simulink model "DISCON_NREL5MW"  (R2016b)
settings: Solver=FixedStepDiscrete  StartTime=0.0  StopTime=inf  FixedStep=Control.DT  RelTol=1e-3
values from neighbouring files (symbols this model uses):
  CertificationSettings =     [Parameters.mat]
  Control =     [Parameters.mat]
  Drivetrain =     [Parameters.mat]
  P_InitAngle = 0.106    [Parameters.mat]
  T_GenSpeedInit = 1104.83    [Parameters.mat]
undefined symbols (not defined in the file or in its folder): DiscIntNeverNeededParam, dLP
settings Model: Creator=evansolingen  LastModifiedBy=sebastiaanmuld
settings DataIOCC: LimitDataPoints=on  SaveFormat=Array  SignalLoggingSaveFormat=ModelDataLogs  SaveOutput=off  SignalLogging=off  SaveTime=off
settings OptimizationCC: ExpressionDepthLimit=2147483647  LifeSpan=inf
settings DebuggingCC: UnderspecifiedInitializationDetection=Classic  MergeDetectMultiDrivingBlocksExec=none  SolverPrmCheckMsg=warning  MultiTaskDSMMsg=warning  MultiTaskCondExecSysMsg=none  FcnCallInpInsideContextMsg=warning  AllowSymbolicDim=off  StateNameClashWarn=warning  SFUnexpectedBacktrackingDiag=warning  SFNoUnconditionalDefaultTransitionDiag=warning  SFExecutionAtInitializationDiag=none
settings HardwareCC: ProdBitPerPointer=32  ProdBitPerSizeT=32  ProdBitPerPtrDiffT=32  ProdLargestAtomicFloat=None  ProdIntDivRoundTo=Undefined  ProdEndianess=Unspecified  ProdWordSize=32  ProdHWDeviceType=32-bit Generic
settings ModelReferenceCC: UpdateModelReferenceTargets=Force  PropagateSignalLabelsOutOfModel=off
settings SFSimCC: SimParseCustomCode=off  SimBuildMode=sf_make_clean
settings RTWCC: SystemTargetFile=discon.tlc  TemplateMakefile=discon_vc.tmf  Description=DISCON DLL Target (for use with GH BLADED)
settings GRTTargetCC: TargetLangStandard=C89/C90 (ANSI)  GeneratePreprocessorConditionals=Disable all  CombineOutputUpdateFcns=off  GRTInterface=on  UseToolchainInfoCompliant=off  ExtModeMexFile=noextcomm
settings ConfigComp: CovMetricSettings=dw  CovHtmlReporting=on  CovSaveCumulativeToWorkspaceVar=on  CovSaveSingleToWorkspaceVar=on  CovExternalEMLEnable=off

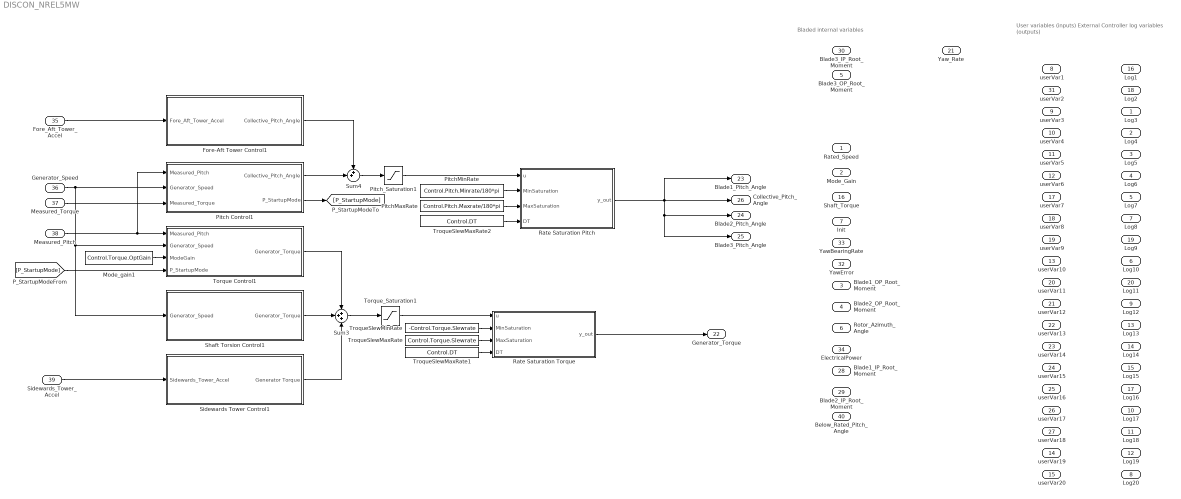
== system DISCON_NREL5MW ==
  note: Bladed internal variables
  note: User variables (inputs)
      | External Controller log variables (outputs)
  Rated_Speed : Inport  PortDimensions=1
  Mode_Gain : Inport  Port=2  PortDimensions=1
  Blade1_OP_Root_Moment : Inport  Port=3  PortDimensions=1
  Blade2_OP_Root_Moment : Inport  Port=4  PortDimensions=1
  Blade3_OP_Root_Moment : Inport  Port=5  PortDimensions=1
  Rotor_Azimuth_Angle : Inport  Port=6  PortDimensions=1
  Init : Inport  Port=7  PortDimensions=1
  userVar1 : Inport  Port=8  PortDimensions=1
  userVar3 : Inport  Port=9  PortDimensions=1
  userVar4 : Inport  Port=10  PortDimensions=1
  userVar5 : Inport  Port=11  PortDimensions=1
  userVar6 : Inport  Port=12  PortDimensions=1
  userVar10 : Inport  Port=13  PortDimensions=1
  userVar19 : Inport  Port=14  PortDimensions=1
  userVar20 : Inport  Port=15  PortDimensions=1
  Shaft_Torque : Inport  Port=16  PortDimensions=1
  userVar7 : Inport  Port=17  PortDimensions=1
  userVar8 : Inport  Port=18  PortDimensions=1
  userVar9 : Inport  Port=19  PortDimensions=1
  userVar11 : Inport  Port=20  PortDimensions=1
  userVar12 : Inport  Port=21  PortDimensions=1
  userVar13 : Inport  Port=22  PortDimensions=1
  userVar14 : Inport  Port=23  PortDimensions=1
  userVar15 : Inport  Port=24  PortDimensions=1
  userVar16 : Inport  Port=25  PortDimensions=1
  userVar17 : Inport  Port=26  PortDimensions=1
  userVar18 : Inport  Port=27  PortDimensions=1
  Blade1_IP_Root_Moment : Inport  Port=28  PortDimensions=1
  Blade2_IP_Root_Moment : Inport  Port=29  PortDimensions=1
  Blade3_IP_Root_Moment : Inport  Port=30  PortDimensions=1
  userVar2 : Inport  Port=31  PortDimensions=1
  YawError : Inport  Port=32  PortDimensions=1
  YawBearingRate : Inport  Port=33  PortDimensions=1
  ElectricalPower : Inport  Port=34  PortDimensions=1
  Fore_Aft_Tower_Accel : Inport  Port=35  PortDimensions=1
  Generator_Speed : Inport  Port=36  PortDimensions=1
  Measured_Torque : Inport  Port=37  PortDimensions=1
  Measured_Pitch : Inport  Port=38  PortDimensions=1
  Sidewards_Tower_Accel : Inport  Port=39  PortDimensions=1
  Below_Rated_Pitch_Angle : Inport  Port=40  PortDimensions=1
  Fore-Aft Tower Control1 : Subsystem
  Mode_gain1 : Constant  Value=Control.Torque.OptGain
  Pitch Control1 : Subsystem
  PitchMaxRate : Constant  Value=Control.Pitch.Maxrate/180*pi
  PitchMinRate : Constant  Value=Control.Pitch.Minrate/180*pi
  Pitch_Saturation1 : Saturate  UpperLimit=Control.Pitch.Max*pi/180  LowerLimit=Control.Pitch.Min*pi/180
  Rate Saturation Pitch : MATLAB Function  TreatAsAtomicUnit=on
  Rate Saturation Torque : MATLAB Function  TreatAsAtomicUnit=on
  Shaft Torsion Control1 : Subsystem
  Sidewards Tower Control1 : Subsystem
  Sum3 : Sum  Inputs=+++
  Sum4 : Sum  Inputs=++|
  Torque Control1 : Subsystem
  Torque_Saturation1 : Saturate  UpperLimit=Control.Torque.Limit  LowerLimit=Control.Torque.Min
  TroqueSlewMaxRate : Constant  Value=Control.Torque.Slewrate
  TroqueSlewMaxRate1 : Constant  Value=Control.DT
  TroqueSlewMaxRate2 : Constant  Value=Control.DT
  TroqueSlewMinRate : Constant  Value=-Control.Torque.Slewrate
  Log3 : Outport  PortDimensions=1
  Log4 : Outport  Port=2  PortDimensions=1
  Log5 : Outport  Port=3  PortDimensions=1
  Log6 : Outport  Port=4  PortDimensions=1
  Log7 : Outport  Port=5  PortDimensions=1
  Log10 : Outport  Port=6  PortDimensions=1
  Log8 : Outport  Port=7  PortDimensions=1
  Log20 : Outport  Port=8  PortDimensions=1
  Log12 : Outport  Port=9  PortDimensions=1
  Log17 : Outport  Port=10  PortDimensions=1
  Log18 : Outport  Port=11  PortDimensions=1
  Log19 : Outport  Port=12  PortDimensions=1
  Log13 : Outport  Port=13  PortDimensions=1
  Log14 : Outport  Port=14  PortDimensions=1
  Log15 : Outport  Port=15  PortDimensions=1
  Log1 : Outport  Port=16  PortDimensions=1
  Log16 : Outport  Port=17  PortDimensions=1
  Log2 : Outport  Port=18  PortDimensions=1
  Log9 : Outport  Port=19  PortDimensions=1
  Log11 : Outport  Port=20  PortDimensions=1
  Yaw_Rate : Outport  Port=21  PortDimensions=1
  Generator_Torque : Outport  Port=22  PortDimensions=1
  Blade1_Pitch_Angle : Outport  Port=23  PortDimensions=1
  Blade2_Pitch_Angle : Outport  Port=24  PortDimensions=1
  Blade3_Pitch_Angle : Outport  Port=25  PortDimensions=1
  Collective_Pitch_Angle : Outport  Port=26  PortDimensions=1
  wires:
  Sidewards_Tower_Accel/1 -> Sidewards Tower Control1/1(Sidewards_Tower_Accel)
  Fore_Aft_Tower_Accel/1 -> Fore-Aft Tower Control1/1(Fore_Aft_Tower_Accel)
  Fore-Aft Tower Control1/1(Collective_Pitch_Angle) -> Sum4/1
  Torque Control1/1(Generator_Torque) -> Sum3/1
  Sidewards Tower Control1/1(Generator Torque) -> Sum3/3
  Measured_Pitch/1 -> Pitch Control1/1(Measured_Pitch), Torque Control1/1(Measured_Pitch)
  Measured_Torque/1 -> Pitch Control1/3(Measured_Torque)
  Shaft Torsion Control1/1(Generator_Torque) -> Sum3/2
  Mode_gain1/1 -> Torque Control1/3(ModeGain)
  Sum3/1 -> Torque_Saturation1/1
  Sum4/1 -> Pitch_Saturation1/1
  Rate Saturation Pitch/1(y_out) -> Blade1_Pitch_Angle/1, Collective_Pitch_Angle/1, Blade3_Pitch_Angle/1, Blade2_Pitch_Angle/1
  PitchMinRate/1 -> Rate Saturation Pitch/2(MinSaturation)
  PitchMaxRate/1 -> Rate Saturation Pitch/3(MaxSaturation)
  Pitch_Saturation1/1 -> Rate Saturation Pitch/1(u)
  Torque_Saturation1/1 -> Rate Saturation Torque/1(u)
  TroqueSlewMinRate/1 -> Rate Saturation Torque/2(MinSaturation)
  TroqueSlewMaxRate/1 -> Rate Saturation Torque/3(MaxSaturation)
  Generator_Speed/1 -> Pitch Control1/2(Generator_Speed), Torque Control1/2(Generator_Speed), Shaft Torsion Control1/1(Generator_Speed)
  [P_StartupMode] -> Torque Control1/4(P_StartupMode)
  Pitch Control1/2(P_StartupMode) -> [P_StartupMode]
  Pitch Control1/1(Collective_Pitch_Angle) -> Sum4/2
  Rate Saturation Torque/1(y_out) -> Generator_Torque/1
  TroqueSlewMaxRate1/1 -> Rate Saturation Torque/4(DT)
  TroqueSlewMaxRate2/1 -> Rate Saturation Pitch/4(DT)

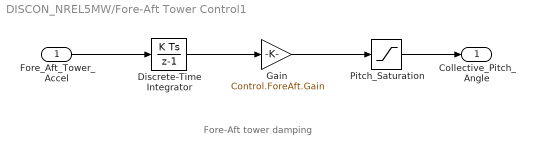
== system DISCON_NREL5MW/Fore-Aft Tower Control1 ==
  note: Fore-Aft tower damping
  Fore_Aft_Tower_Accel : Inport
  Discrete-Time Integrator : DiscreteIntegrator  SampleTime=-1  ICPrevOutput=DiscIntNeverNeededParam  ICPrevScaledInput=DiscIntNeverNeededParam
  Gain : Gain  Gain=Control.ForeAft.Gain
  Pitch_Saturation : Saturate  UpperLimit=Control.ForeAft.MaxPitchAmplitude*pi/180  LowerLimit=-Control.ForeAft.MaxPitchAmplitude*pi/180
  Collective_Pitch_Angle : Outport
  wires:
  Fore_Aft_Tower_Accel/1 -> Discrete-Time Integrator/1
  Pitch_Saturation/1 -> Collective_Pitch_Angle/1
  Discrete-Time Integrator/1 -> Gain/1
  Gain/1 -> Pitch_Saturation/1

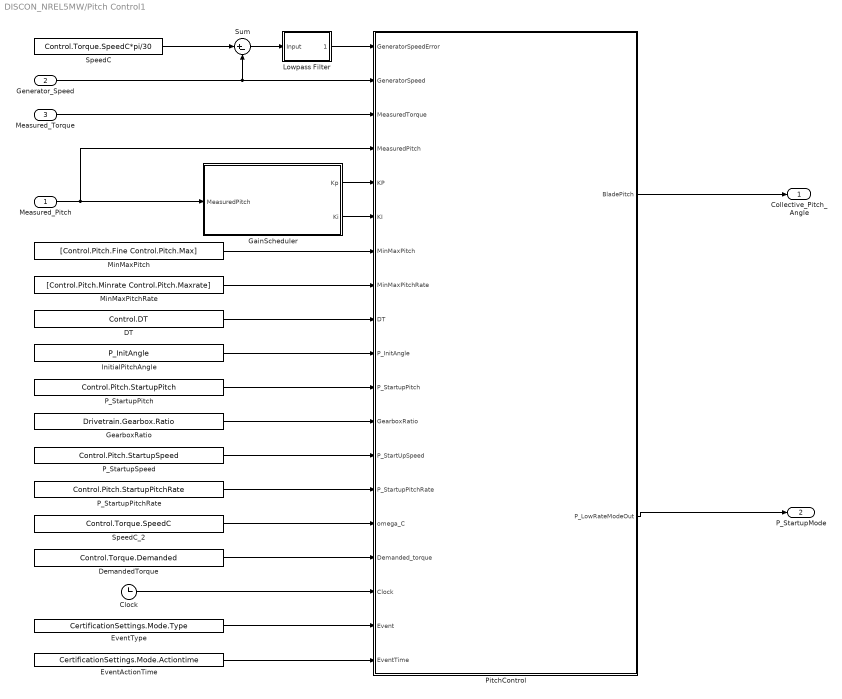
== system DISCON_NREL5MW/Pitch Control1 ==
  Measured_Pitch : Inport
  Generator_Speed : Inport  Port=2
  Measured_Torque : Inport  Port=3
  Clock : Clock
  DT : Constant  Value=Control.DT
  DemandedTorque : Constant  Value=Control.Torque.Demanded
  EventActionTime : Constant  Value=CertificationSettings.Mode.Actiontime
  EventType : Constant  Value=CertificationSettings.Mode.Type
  GainScheduler : Subsystem
  GearboxRatio : Constant  Value=Drivetrain.Gearbox.Ratio
  InitialPitchAngle : Constant  Value=P_InitAngle
  Lowpass Filter : Subsystem
  MinMaxPitch : Constant  Value=[Control.Pitch.Fine Control.Pitch.Max]
  MinMaxPitchRate : Constant  Value=[Control.Pitch.Minrate Control.Pitch.Maxrate]
  P_StartupPitch : Constant  Value=Control.Pitch.StartupPitch
  P_StartupPitchRate : Constant  Value=Control.Pitch.StartupPitchRate
  P_StartupSpeed : Constant  Value=Control.Pitch.StartupSpeed
  PitchControl : MATLAB Function  TreatAsAtomicUnit=on
  SpeedC : Constant  Value=Control.Torque.SpeedC*pi/30
  SpeedC_2 : Constant  Value=Control.Torque.SpeedC
  Sum : Sum  Inputs=|+-
  Collective_Pitch_Angle : Outport
  P_StartupMode : Outport  Port=2
  wires:
  MinMaxPitch/1 -> PitchControl/7(MinMaxPitch)
  MinMaxPitchRate/1 -> PitchControl/8(MinMaxPitchRate)
  PitchControl/1(BladePitch) -> Collective_Pitch_Angle/1
  Measured_Torque/1 -> PitchControl/3(MeasuredTorque)
  SpeedC/1 -> Sum/1
  Generator_Speed/1 -> PitchControl/2(GeneratorSpeed), Sum/2
  Sum/1 -> Lowpass Filter/1(Input)
  Lowpass Filter/1(Output) -> PitchControl/1(GeneratorSpeedError)
  PitchControl/2(P_LowRateModeOut) -> P_StartupMode/1
  DT/1 -> PitchControl/9(DT)
  P_StartupPitch/1 -> PitchControl/11(P_StartupPitch)
  InitialPitchAngle/1 -> PitchControl/10(P_InitAngle)
  GearboxRatio/1 -> PitchControl/12(GearboxRatio)
  P_StartupSpeed/1 -> PitchControl/13(P_StartUpSpeed)
  P_StartupPitchRate/1 -> PitchControl/14(P_StartupPitchRate)
  SpeedC_2/1 -> PitchControl/15(omega_C)
  DemandedTorque/1 -> PitchControl/16(Demanded_torque)
  Measured_Pitch/1 -> PitchControl/4(MeasuredPitch), GainScheduler/1(MeasuredPitch)
  EventType/1 -> PitchControl/18(Event)
  Clock/1 -> PitchControl/17(Clock)
  EventActionTime/1 -> PitchControl/19(EventTime)
  GainScheduler/1(Kp) -> PitchControl/5(KP)
  GainScheduler/2(Ki) -> PitchControl/6(KI)

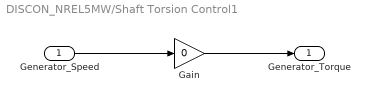
== system DISCON_NREL5MW/Shaft Torsion Control1 ==
  Generator_Speed : Inport
  Gain : Gain  Gain=0
  Generator_Torque : Outport
  wires:
  Generator_Speed/1 -> Gain/1
  Gain/1 -> Generator_Torque/1

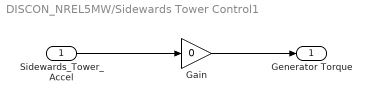
== system DISCON_NREL5MW/Sidewards Tower Control1 ==
  Sidewards_Tower_Accel : Inport
  Gain : Gain  Gain=0
  Generator Torque : Outport
  wires:
  Sidewards_Tower_Accel/1 -> Gain/1
  Gain/1 -> Generator Torque/1

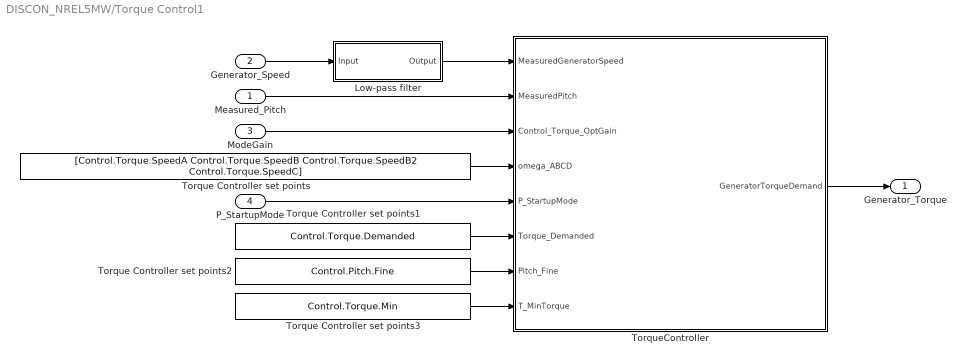
== system DISCON_NREL5MW/Torque Control1 ==
  Measured_Pitch : Inport
  Generator_Speed : Inport  Port=2
  ModeGain : Inport  Port=3
  P_StartupMode : Inport  Port=4
  Low-pass filter : Subsystem
  Torque Controller set points : Constant  Value=[Control.Torque.SpeedA Control.Torque.SpeedB Control.Torque.SpeedB2 Control.Torque.SpeedC]
  Torque Controller set points1 : Constant  Value=Control.Torque.Demanded
  Torque Controller set points2 : Constant  Value=Control.Pitch.Fine
  Torque Controller set points3 : Constant  Value=Control.Torque.Min
  TorqueController : MATLAB Function  TreatAsAtomicUnit=on
  Generator_Torque : Outport
  wires:
  Generator_Speed/1 -> Low-pass filter/1(Input)
  TorqueController/1(GeneratorTorqueDemand) -> Generator_Torque/1
  Measured_Pitch/1 -> TorqueController/2(MeasuredPitch)
  ModeGain/1 -> TorqueController/3(Control_Torque_OptGain)
  Torque Controller set points/1 -> TorqueController/4(omega_ABCD)
  P_StartupMode/1 -> TorqueController/5(P_StartupMode)
  Low-pass filter/1(Output) -> TorqueController/1(MeasuredGeneratorSpeed)
  Torque Controller set points3/1 -> TorqueController/8(T_MinTorque)
  Torque Controller set points2/1 -> TorqueController/7(Pitch_Fine)
  Torque Controller set points1/1 -> TorqueController/6(Torque_Demanded)

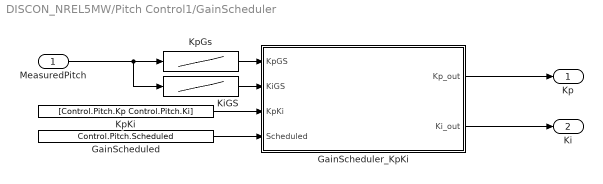
== system DISCON_NREL5MW/Pitch Control1/GainScheduler ==
  MeasuredPitch : Inport
  GainScheduled : Constant  Value=Control.Pitch.Scheduled
  GainScheduler_KpKi : MATLAB Function  TreatAsAtomicUnit=on
  KiGS : Lookup_n-D  NumberOfTableDimensions=1  BreakpointsForDimension1=Control.Pitch.ScheduledPitchAngles  Table=Control.Pitch.KiGS  ExtrapMethod=Clip  UseLastTableValue=on  InternalRulePriority=Speed  RndMeth=Simplest  InputSameDT=on
  KpGs : Lookup_n-D  NumberOfTableDimensions=1  BreakpointsForDimension1=Control.Pitch.ScheduledPitchAngles  Table=Control.Pitch.KpGS  ExtrapMethod=Clip  UseLastTableValue=on  InternalRulePriority=Speed  RndMeth=Simplest  InputSameDT=on
  KpKi : Constant  Value=[Control.Pitch.Kp Control.Pitch.Ki]
  Kp : Outport
  Ki : Outport  Port=2
  wires:
  MeasuredPitch/1 -> KiGS/1, KpGs/1
  GainScheduled/1 -> GainScheduler_KpKi/4(Scheduled)
  GainScheduler_KpKi/2(Ki_out) -> Ki/1
  KpKi/1 -> GainScheduler_KpKi/3(KpKi)
  KpGs/1 -> GainScheduler_KpKi/1(KpGS)
  KiGS/1 -> GainScheduler_KpKi/2(KiGS)
  GainScheduler_KpKi/1(Kp_out) -> Kp/1

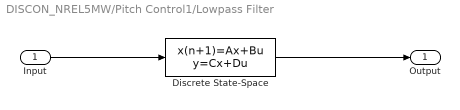
== system DISCON_NREL5MW/Pitch Control1/Lowpass Filter ==
  Input : Inport
  Discrete State-Space : DiscreteStateSpace  A=dLP.a  B=dLP.b  C=dLP.c  D=dLP.d  SampleTime=-1
  Output : Outport
  wires:
  Input/1 -> Discrete State-Space/1
  Discrete State-Space/1 -> Output/1

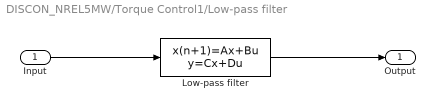
== system DISCON_NREL5MW/Torque Control1/Low-pass filter ==
  Input : Inport
  Low-pass filter : DiscreteStateSpace  A=dLP.a  B=dLP.b  C=dLP.c  D=dLP.d  X0=T_GenSpeedInit*(pi/30)/dLP.c  SampleTime=-1
  Output : Outport
  wires:
  Input/1 -> Low-pass filter/1
  Low-pass filter/1 -> Output/1

== matlab function DISCON_NREL5MW/Rate Saturation Pitch ==
  data: u input; MinSaturation input; y_out output; MaxSaturation input; DT input
function y_out = fcn(u, MinSaturation, MaxSaturation, DT)
persistent y

if isempty(y)
    y = u;
end

rate = (u-y)/DT;
rate = min(max(rate, MinSaturation), MaxSaturation);

y = y + rate*DT;
y_out = y;

== matlab function DISCON_NREL5MW/Pitch Control1/PitchControl ==
  settings: sampleTime=Control.DT
  data: GeneratorSpeedError input; GeneratorSpeed input; MeasuredTorque input; MeasuredPitch input; BladePitch output; KP input; KI input; MinMaxPitch input; MinMaxPitchRate input; DT input; P_InitAngle input; P_StartupPitch input; GearboxRatio input; P_StartUpSpeed input; P_StartupPitchRate input; omega_C input; Demanded_torque input; Clock input; P_LowRateModeOut output; Event input; EventTime input
function [BladePitch, P_LowRateModeOut]  = PitchControl(GeneratorSpeedError, GeneratorSpeed, MeasuredTorque, MeasuredPitch, KP, KI, MinMaxPitch, MinMaxPitchRate, DT, P_InitAngle, P_StartupPitch, GearboxRatio, P_StartUpSpeed, P_StartupPitchRate, omega_C, Demanded_torque, Clock, Event, EventTime)
persistent I_term PI_term_old P_LowRateMode P_LowRateMode_old

%Initialize all persistent variables
if isempty(I_term)
    I_term = (P_InitAngle*pi/180);
    PI_term_old = (P_InitAngle*pi/180);
    P_LowRateMode = true;
    P_LowRateMode_old = true; %Used to detect change from start-up/below-rated to above-rated operation mode
end

%Event handling part
if (Event == 2 && Clock >= EventTime) || (Event == 5 && Clock >= EventTime) %Grid loss, emergency shutdown
    P_LowRateMode = false;
    P_MinPitchSat = MinMaxPitch(2)*pi/180;
elseif (Event == 4 && Clock >= EventTime) % Normal shutdown
    P_LowRateMode = true;
    P_MinPitchSat = MinMaxPitch(2)*pi/180;
elseif Event == 7 || Event == 6 % Idling and parked mode
    P_MinPitchSat = MinMaxPitch(2)*pi/180;
elseif MeasuredTorque > Demanded_torque*0.99 || GeneratorSpeed > omega_C*(pi/30) % Above-rated operating mode
    P_LowRateMode = false;
    P_MinPitchSat = MinMaxPitch(1)*pi/180;
    if P_LowRateMode ~= P_LowRateMode_old % On switching event between below-rated to above rated, reinitialize the integral term to ensure smooth transition
        I_term = MeasuredPitch;
    end
elseif Event == 3 || GeneratorSpeed < P_StartUpSpeed*GearboxRatio*(pi/30) % Normal startup 
    if Event == 3 && Clock < EventTime
        P_LowRateMode = true;
        P_MinPitchSat = MinMaxPitch(2)*pi/180;
    elseif (Event == 3 && Clock >= EventTime) && (GeneratorSpeed < P_StartUpSpeed*GearboxRatio*(pi/30))
        P_LowRateMode = true;
        P_MinPitchSat = P_StartupPitch*pi/180;
    else
        P_LowRateMode = true;
        P_MinPitchSat = MinMaxPitch(1)*pi/180;
    end
else
    P_MinPitchSat = MinMaxPitch(1)*pi/180;
end
 
% Pitch controller, KP and KI are constant or gain-scheduled, depending on
% input. Integral term is saturated, lower bound is variable and depends on
% event or operatinig mode.
P_term = KP*GeneratorSpeedError;
I_term = I_term + KI*GeneratorSpeedError*DT;
I_term = min(max(I_term,P_MinPitchSat), MinMaxPitch(2)*pi/180);

PI_term = P_term + I_term;
PI_term_sat = min(max(PI_term,P_MinPitchSat), MinMaxPitch(2)*pi/180);

% Calculate and limit pitch rate. Limit on rate is subject to event or
% operating mode.
PitchRate = (PI_term_sat - PI_term_old)/DT;
if P_LowRateMode
    PitchRate = min(max(PitchRate, -P_StartupPitchRate*pi/180), P_StartupPitchRate*pi/180);
else
    PitchRate = min(max(PitchRate, MinMaxPitchRate(1)*pi/180), MinMaxPitchRate(2)*pi/180);
end
BladePitch = PI_term_old + PitchRate*DT;

% Write variables to persistent variables and/or outputs
PI_term_old = BladePitch;
P_LowRateModeOut = P_LowRateMode;
P_LowRateMode_old = P_LowRateMode;
end

== matlab function DISCON_NREL5MW/Pitch Control1/GainScheduler/GainScheduler_KpKi ==
  data: KpGS input; KiGS input; Kp_out output; KpKi input; Scheduled input; Ki_out output
function [Kp_out, Ki_out] = fcn(KpGS, KiGS, KpKi, Scheduled)

if Scheduled > 0.5
    Kp_out = KpGS;
    Ki_out = KiGS;
else
    Kp_out = KpKi(1);
    Ki_out = KpKi(2);
end

== matlab function DISCON_NREL5MW/Rate Saturation Torque ==
  data: u input; MinSaturation input; y_out output; MaxSaturation input; DT input
function y_out = fcn(u, MinSaturation, MaxSaturation, DT)
persistent y

if isempty(y)
    y = u;
end

rate = (u-y)/DT;
rate = min(max(rate, MinSaturation), MaxSaturation);

y = y + rate*DT;
y_out = y;

== matlab function DISCON_NREL5MW/Torque Control1/TorqueController ==
  data: GeneratorTorqueDemand output; MeasuredGeneratorSpeed input; MeasuredPitch input; Control_Torque_OptGain input; omega_ABCD input size=[1 4]; P_StartupMode input; Torque_Demanded input; Pitch_Fine input; T_MinTorque input
function GeneratorTorqueDemand  = TorqueController(MeasuredGeneratorSpeed, MeasuredPitch, Control_Torque_OptGain, omega_ABCD, P_StartupMode, Torque_Demanded, Pitch_Fine, T_MinTorque)

% Calculate generator torque setpoint according to the feedforward wind
% turbine control law T = K*\omega^2
GeneratorTorqueDemand = max(min(Control_Torque_OptGain*MeasuredGeneratorSpeed^2, Torque_Demanded), T_MinTorque);

% Calculate torques at beginning and end of CP_max operation
TorqueOmegaB = Control_Torque_OptGain*(omega_ABCD(2)*pi/30)^2;
TorqueOmegaC = Control_Torque_OptGain*(omega_ABCD(3)*pi/30)^2;

% Apply maximum demanded torque when pitch is 1 degree above fine-pitch and
% the wind turbine is not in start-up mode.
if MeasuredPitch > (Pitch_Fine + .1)*pi/180 && P_StartupMode == false
    GeneratorTorqueDemand = Torque_Demanded;
elseif MeasuredGeneratorSpeed < omega_ABCD(1)*pi/30
    GeneratorTorqueDemand = T_MinTorque;
elseif MeasuredGeneratorSpeed < omega_ABCD(2)*pi/30
    GeneratorTorqueDemand = (TorqueOmegaB - T_MinTorque)/((omega_ABCD(2) - omega_ABCD(1))*pi/30)*(MeasuredGeneratorSpeed - omega_ABCD(1)*pi/30) + T_MinTorque;
elseif MeasuredGeneratorSpeed >= omega_ABCD(3)*pi/30
    GeneratorTorqueDemand = (Torque_Demanded - TorqueOmegaC)/((omega_ABCD(4) - omega_ABCD(3))*pi/30)*(MeasuredGeneratorSpeed - omega_ABCD(3)*pi/30) + TorqueOmegaC;
end
